simulink model "PID2"  (R2022b)
settings: Solver=FixedStepAuto  StartTime=0.0  StopTime=150  FixedStep=0.01  RelTol=1e-3
settings Model: Creator=giuli  LastModifiedBy=giuli

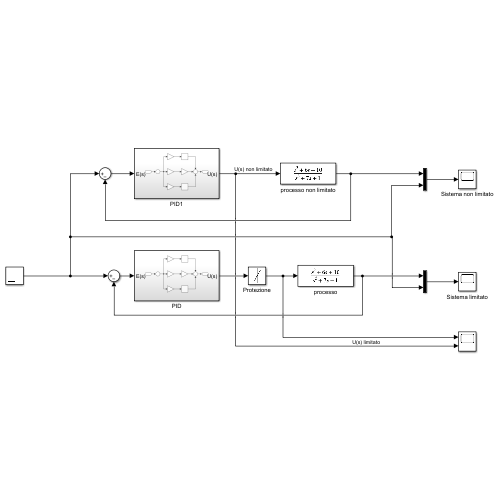
[thumbnail: Simulink's stored preview of the top-level diagram]
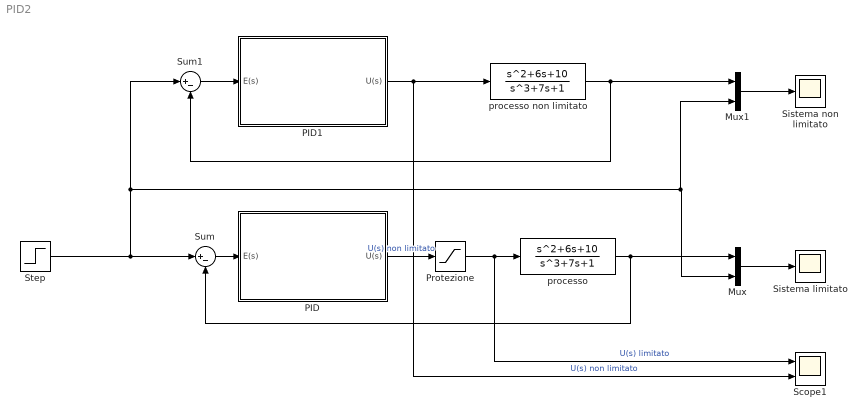
== system PID2 ==
  Mux : Mux  Inputs=2
  Mux1 : Mux  Inputs=2
  PID : Subsystem
  PID1 : Subsystem
  Protezione : Saturate  UpperLimit=5  LowerLimit=-5
  Scope1 : Scope  NumInputPorts=2
  Sistema limitato : Scope
  Sistema non limitato : Scope
  Step : Step  Time=5  SampleTime=0
  Sum : Sum  Inputs=|+-
  Sum1 : Sum  Inputs=|+-
  processo : TransferFcn  Numerator=[1 6 10]  Denominator=[1 0 7 1]
  processo non limitato : TransferFcn  Numerator=[1 6 10]  Denominator=[1 0 7 1]
  wires:
  Step/1 -> Sum/1, Sum1/1, Mux1/2, Mux/2
  processo/1 -> Mux/1, Sum/2
  Mux/1 -> Sistema limitato/1
  PID/1(U(s)) -> Protezione/1  "U(s) non limitato"
  Sum/1 -> PID/1(E(s))
  Protezione/1 -> Scope1/1, processo/1  "U(s) limitato"
  Mux1/1 -> Sistema non limitato/1
  processo non limitato/1 -> Sum1/2, Mux1/1
  PID1/1(U(s)) -> Scope1/2, processo non limitato/1  "U(s) non limitato"
  Sum1/1 -> PID1/1(E(s))

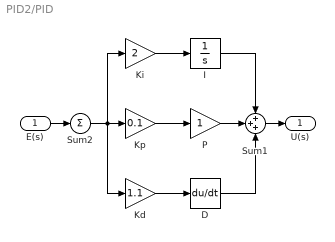
== system PID2/PID ==
  E(s) : Inport
  D : Derivative
  I : Integrator
  Kd : Gain  Gain=1.1
  Ki : Gain  Gain=2
  Kp : Gain  Gain=0.1
  P : Gain
  Sum1 : Sum  Inputs=+++
  Sum2 : Sum  Inputs=+
  U(s) : Outport
  wires:
  Sum2/1 -> Kp/1, Kd/1, Ki/1
  I/1 -> Sum1/1
  Sum1/1 -> U(s)/1
  D/1 -> Sum1/3
  P/1 -> Sum1/2
  E(s)/1 -> Sum2/1
  Ki/1 -> I/1
  Kp/1 -> P/1
  Kd/1 -> D/1

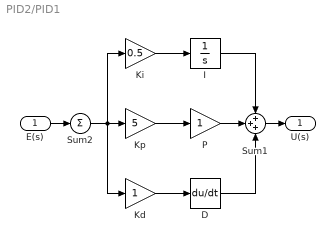
== system PID2/PID1 ==
  E(s) : Inport
  D : Derivative
  I : Integrator
  Kd : Gain
  Ki : Gain  Gain=0.5
  Kp : Gain  Gain=5
  P : Gain
  Sum1 : Sum  Inputs=+++
  Sum2 : Sum  Inputs=+
  U(s) : Outport
  wires:
  Kd/1 -> D/1
  Kp/1 -> P/1
  Ki/1 -> I/1
  E(s)/1 -> Sum2/1
  P/1 -> Sum1/2
  D/1 -> Sum1/3
  Sum1/1 -> U(s)/1
  I/1 -> Sum1/1
  Sum2/1 -> Ki/1, Kd/1, Kp/1
